simulink model "special_ports"  (R2014a)
settings: Solver=ode45  StartTime=0.0  StopTime=10.0  RelTol=1e-3
settings Model: Creator=ladmin  LastModifiedBy=ladmin

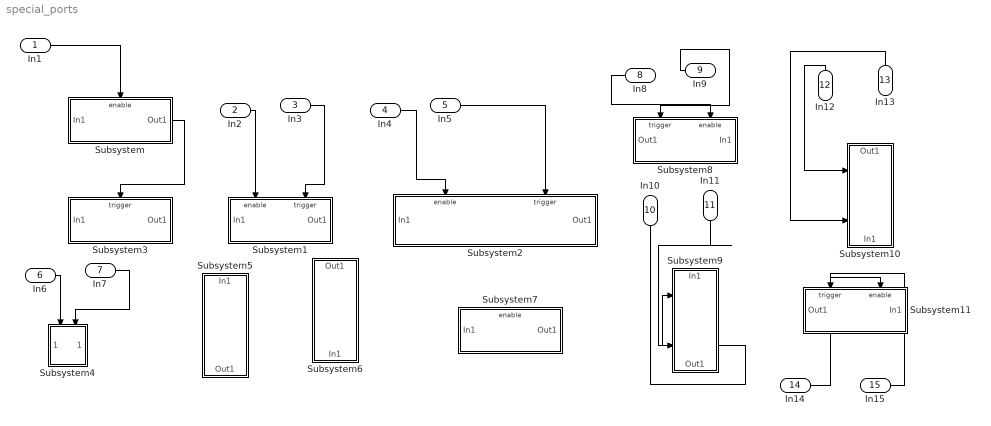
== system special_ports ==
  In1 : Inport
  In2 : Inport  Port=2
  In3 : Inport  Port=3
  In4 : Inport  Port=4
  In5 : Inport  Port=5
  In6 : Inport  Port=6
  In7 : Inport  Port=7
  In8 : Inport  Port=8
  In9 : Inport  Port=9
  In10 : Inport  Port=10
  In11 : Inport  Port=11
  In12 : Inport  Port=12
  In13 : Inport  Port=13
  In14 : Inport  Port=14
  In15 : Inport  Port=15
  Subsystem : Subsystem
  Subsystem1 : Subsystem
  Subsystem10 : Subsystem
  Subsystem11 : Subsystem
  Subsystem2 : Subsystem
  Subsystem3 : Subsystem
  Subsystem4 : Subsystem
  Subsystem5 : Subsystem
  Subsystem6 : Subsystem
  Subsystem7 : Subsystem
  Subsystem8 : Subsystem
  Subsystem9 : Subsystem
  wires:
  Subsystem/1(Out1) -> Subsystem3/Trigger
  In1/1 -> Subsystem/Enable
  In2/1 -> Subsystem1/Enable
  In3/1 -> Subsystem1/Trigger
  In4/1 -> Subsystem2/Enable
  In5/1 -> Subsystem2/Trigger
  In6/1 -> Subsystem4/Enable
  In7/1 -> Subsystem4/Trigger
  In8/1 -> Subsystem8/Enable
  In9/1 -> Subsystem8/Trigger
  In10/1 -> Subsystem9/Enable
  In11/1 -> Subsystem9/Trigger
  In12/1 -> Subsystem10/Enable
  In13/1 -> Subsystem10/Trigger
  In14/1 -> Subsystem11/Enable
  In15/1 -> Subsystem11/Trigger

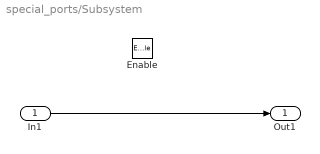
== system special_ports/Subsystem ==
  In1 : Inport
  Enable : EnablePort
  Out1 : Outport
  wires:
  In1/1 -> Out1/1

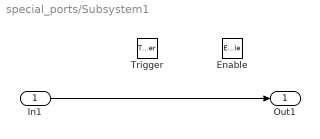
== system special_ports/Subsystem1 ==
  In1 : Inport
  Enable : EnablePort
  Trigger : TriggerPort  PortDimensions=1
  Out1 : Outport
  wires:
  In1/1 -> Out1/1

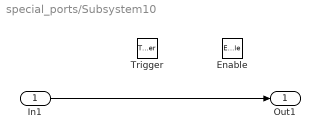
== system special_ports/Subsystem10 ==
  In1 : Inport
  Enable : EnablePort
  Trigger : TriggerPort  PortDimensions=1
  Out1 : Outport
  wires:
  In1/1 -> Out1/1

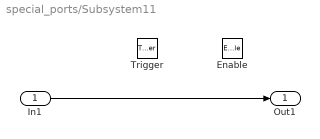
== system special_ports/Subsystem11 ==
  In1 : Inport
  Enable : EnablePort
  Trigger : TriggerPort  PortDimensions=1
  Out1 : Outport
  wires:
  In1/1 -> Out1/1

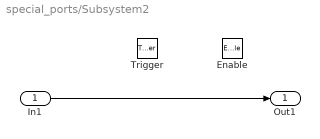
== system special_ports/Subsystem2 ==
  In1 : Inport
  Enable : EnablePort
  Trigger : TriggerPort  PortDimensions=1
  Out1 : Outport
  wires:
  In1/1 -> Out1/1

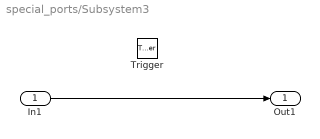
== system special_ports/Subsystem3 ==
  In1 : Inport
  Trigger : TriggerPort  PortDimensions=1
  Out1 : Outport
  wires:
  In1/1 -> Out1/1

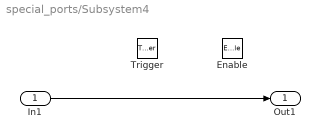
== system special_ports/Subsystem4 ==
  In1 : Inport
  Enable : EnablePort
  Trigger : TriggerPort  PortDimensions=1
  Out1 : Outport
  wires:
  In1/1 -> Out1/1

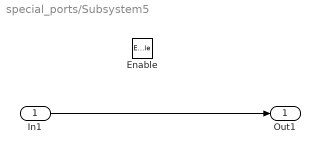
== system special_ports/Subsystem5 ==
  In1 : Inport
  Enable : EnablePort
  Out1 : Outport
  wires:
  In1/1 -> Out1/1

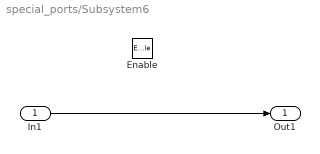
== system special_ports/Subsystem6 ==
  In1 : Inport
  Enable : EnablePort
  Out1 : Outport
  wires:
  In1/1 -> Out1/1

== system special_ports/Subsystem7 ==
  In1 : Inport
  Enable : EnablePort
  Out1 : Outport
  wires:
  In1/1 -> Out1/1

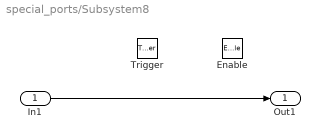
== system special_ports/Subsystem8 ==
  In1 : Inport
  Enable : EnablePort
  Trigger : TriggerPort  PortDimensions=1
  Out1 : Outport
  wires:
  In1/1 -> Out1/1

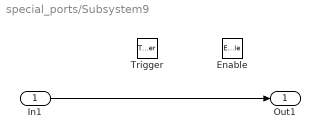
== system special_ports/Subsystem9 ==
  In1 : Inport
  Enable : EnablePort
  Trigger : TriggerPort  PortDimensions=1
  Out1 : Outport
  wires:
  In1/1 -> Out1/1
